simulink model "HYBRID_CONTROLLER"  (R2022b)
settings: Solver=FixedStepAuto  StartTime=0.0  StopTime=200  FixedStep=0.1  RelTol=1e-3
values from neighbouring files (symbols this model uses):
  trajectory = generateTimedTrajectory(smoothed_waypoints, time_waypoints,                                         actual_duration, time_vector, L)    [generateImprovedTrajectory.m]
undefined symbols (not defined in the file or in its folder): controller_params
libraries: robotmobilelib x1
settings Model: Creator=emanuela  LastModifiedBy=emanuela
settings DataIOCC: ReturnWorkspaceOutputs=off

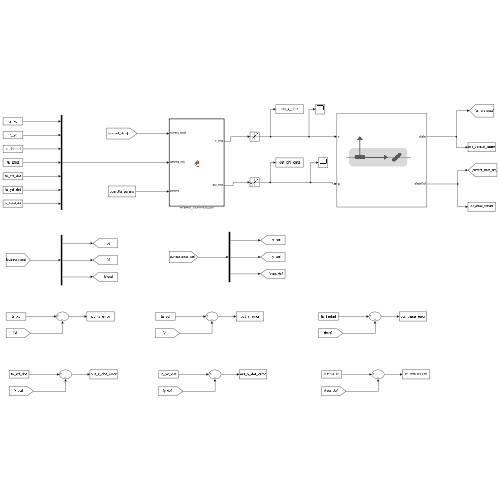
[thumbnail: Simulink's stored preview of the top-level diagram]
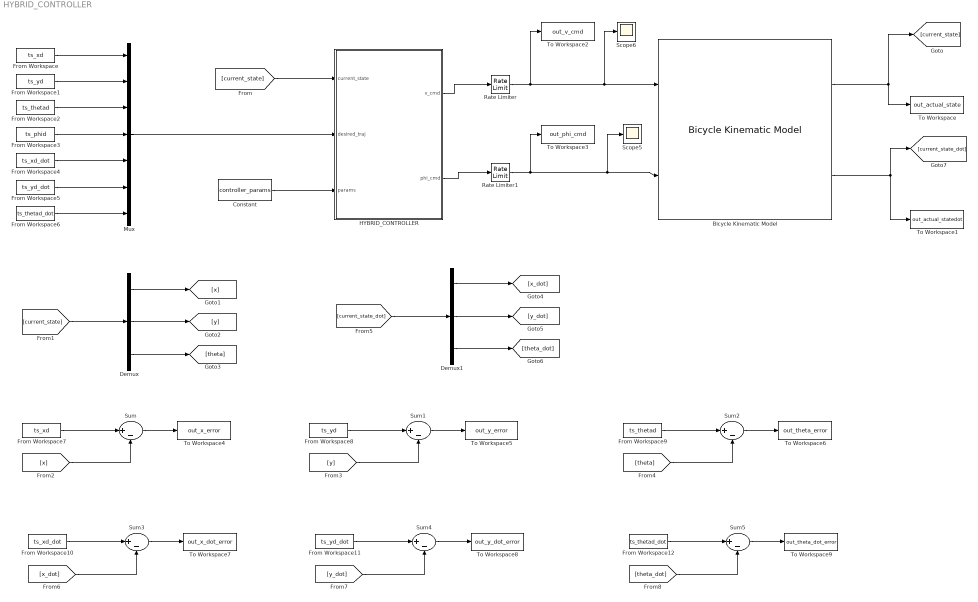
== system HYBRID_CONTROLLER ==
  Bicycle Kinematic Model : robotmobilelib/Bicycle Kinematic Model  VehicleInputs=Vehicle Speed & Steering Angle  WheelBase=2.8  VehicleSpeedRange=[0 3]  MaxSteeringAngle=pi/4  InitialState=[trajectory.xd(1), trajectory.yd(1), trajectory.thetad(1)]  SimulateUsing=Interpreted execution
  Constant : Constant  Value=controller_params  OutDataTypeStr=Bus: controller_params_bus
  Demux : Demux  Outputs=3
  Demux1 : Demux  Outputs=3
  From Workspace : FromWorkspace  VariableName=ts_xd
  From Workspace1 : FromWorkspace  VariableName=ts_yd
  From Workspace10 : FromWorkspace  VariableName=ts_xd_dot
  From Workspace11 : FromWorkspace  VariableName=ts_yd_dot
  From Workspace12 : FromWorkspace  VariableName=ts_thetad_dot
  From Workspace2 : FromWorkspace  VariableName=ts_thetad
  From Workspace3 : FromWorkspace  VariableName=ts_phid
  From Workspace4 : FromWorkspace  VariableName=ts_xd_dot
  From Workspace5 : FromWorkspace  VariableName=ts_yd_dot
  From Workspace6 : FromWorkspace  VariableName=ts_thetad_dot
  From Workspace7 : FromWorkspace  VariableName=ts_xd
  From Workspace8 : FromWorkspace  VariableName=ts_yd
  From Workspace9 : FromWorkspace  VariableName=ts_thetad
  HYBRID_CONTROLLER : MATLAB Function  TreatAsAtomicUnit=on
  Mux : Mux  Inputs=7
  Rate Limiter : RateLimiter  SampleTimeMode=inherited
  Rate Limiter1 : RateLimiter  SampleTimeMode=inherited
  Scope5 : Scope
  Scope6 : Scope
  Sum{,1..5} (6 alike) : Sum  Inputs=|+-
  To Workspace : ToWorkspace  VariableName=out_actual_state  SaveFormat=Timeseries  SampleTime=-1
  To Workspace1 : ToWorkspace  VariableName=out_actual_statedot  SaveFormat=Timeseries  SampleTime=-1
  To Workspace2 : ToWorkspace  VariableName=out_v_cmd  SaveFormat=Timeseries  SampleTime=-1
  To Workspace3 : ToWorkspace  VariableName=out_phi_cmd  SaveFormat=Timeseries  SampleTime=-1
  To Workspace4 : ToWorkspace  VariableName=out_x_error  SaveFormat=Timeseries  SampleTime=-1
  To Workspace5 : ToWorkspace  VariableName=out_y_error  SaveFormat=Timeseries  SampleTime=-1
  To Workspace6 : ToWorkspace  VariableName=out_theta_error  SaveFormat=Timeseries  SampleTime=-1
  To Workspace7 : ToWorkspace  VariableName=out_x_dot_error  SaveFormat=Timeseries  SampleTime=-1
  To Workspace8 : ToWorkspace  VariableName=out_y_dot_error  SaveFormat=Timeseries  SampleTime=-1
  To Workspace9 : ToWorkspace  VariableName=out_theta_dot_error  SaveFormat=Timeseries  SampleTime=-1
  wires:
  HYBRID_CONTROLLER/2(phi_cmd) -> Rate Limiter1/1
  HYBRID_CONTROLLER/1(v_cmd) -> Rate Limiter/1
  Constant/1 -> HYBRID_CONTROLLER/3(params)
  From Workspace4/1 -> Mux/5
  From Workspace/1 -> Mux/1
  From Workspace1/1 -> Mux/2
  From Workspace2/1 -> Mux/3
  From Workspace3/1 -> Mux/4
  From Workspace5/1 -> Mux/6
  From Workspace6/1 -> Mux/7
  Bicycle Kinematic Model/1 -> To Workspace/1, [current_state]
  Bicycle Kinematic Model/2 -> To Workspace1/1, [current_state_dot]
  Mux/1 -> HYBRID_CONTROLLER/2(desired_traj)
  [current_state] -> HYBRID_CONTROLLER/1(current_state)
  [current_state] -> Demux/1
  Demux/1 -> [x]
  Demux/2 -> [y]
  Demux/3 -> [theta]
  [x] -> Sum/2
  From Workspace7/1 -> Sum/1
  Sum/1 -> To Workspace4/1
  From Workspace8/1 -> Sum1/1
  Sum1/1 -> To Workspace5/1
  [y] -> Sum1/2
  [theta] -> Sum2/2
  Sum2/1 -> To Workspace6/1
  From Workspace9/1 -> Sum2/1
  [current_state_dot] -> Demux1/1
  Demux1/1 -> [x_dot]
  Demux1/2 -> [y_dot]
  Demux1/3 -> [theta_dot]
  [theta_dot] -> Sum5/2
  Sum5/1 -> To Workspace9/1
  From Workspace10/1 -> Sum3/1
  From Workspace11/1 -> Sum4/1
  [y_dot] -> Sum4/2
  Sum4/1 -> To Workspace8/1
  From Workspace12/1 -> Sum5/1
  Sum3/1 -> To Workspace7/1
  [x_dot] -> Sum3/2
  Rate Limiter/1 -> To Workspace2/1, Scope6/1, Bicycle Kinematic Model/1
  Rate Limiter1/1 -> To Workspace3/1, Scope5/1, Bicycle Kinematic Model/2

== matlab function HYBRID_CONTROLLER/HYBRID_CONTROLLER ==
  settings: updateMethod=DISCRETE  sampleTime=0.1
  data: current_state input; v_cmd output; desired_traj input; params input; phi_cmd output
function [v_cmd, phi_cmd] = fcn(current_state, desired_traj, params)
    [v_cmd, phi_cmd] = Hybrid_Controller(current_state, desired_traj, params);
end
